simulink model "s0416"  (Simulink 7.0)
settings: Solver=ode3  SolverMode=SingleTasking  StartTime=0.0  StopTime=900  FixedStep=1  MaxStep=1  RelTol=1e-3  AbsTol=1e-6
values from neighbouring files (symbols this model uses):
  Kpr = 10    [m0108d.m]    (also in m0109b.m = 1; m0113c.m; m0404Bsp.m = 3)
  t0A = -1    [m0404Bsp.m]
undefined symbols (not defined in the file or in its folder): eAdach, edach, T1D, Tv
settings Model: Creator=froriep  LastModifiedBy=froriep
settings DataIOCC: LimitDataPoints=off  SaveOutput=off  SaveTime=off
settings OptimizationCC: BooleanDataType=off
settings DebuggingCC: SaveWithParameterizedLinksMsg=none  SignalResolutionControl=TryResolveAllWithWarning  SolverPrmCheckMsg=none  MultiTaskDSMMsg=warning  MultiTaskCondExecSysMsg=none  StrictBusMsg=None
settings HardwareCC: TargetUnknown=on
settings RTWCC: IncludeERTFirstTime=on

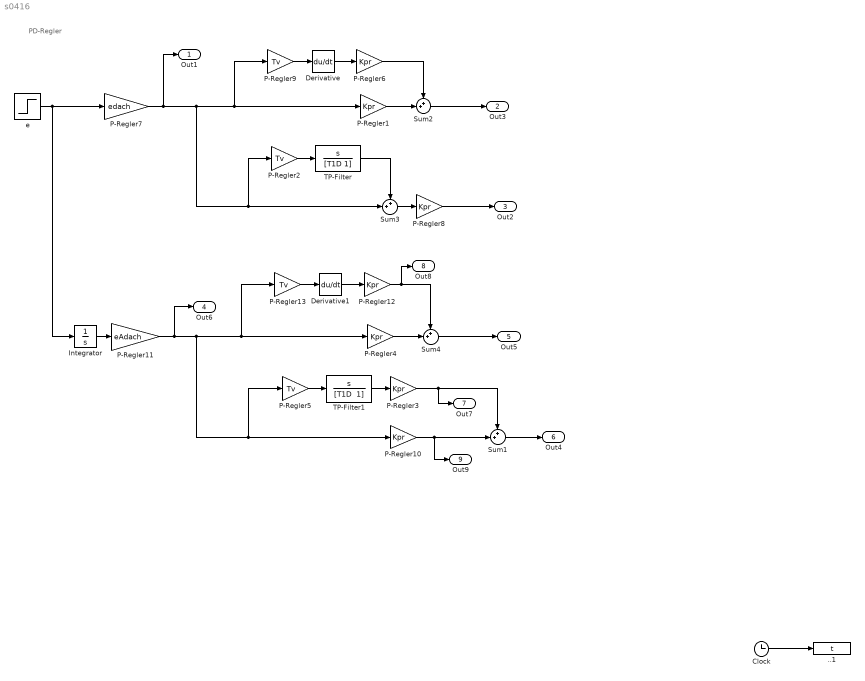
== system s0416 ==
  note: PD-Regler
  ..1 : ToWorkspace  VariableName=t  SaveFormat=Array
  Clock : Clock
      settings: Decimation=10
  Derivative : Derivative
  Derivative1 : Derivative
  Integrator : Integrator
  P-Regler{1,3..4,6,8,10,12} (7 alike) : Gain  Gain=Kpr  ParameterDataType=sfix(16)  ParameterScaling=2^0  OutDataType=sfix(16)  OutScaling=2^0
  P-Regler11 : Gain  Gain=eAdach  ParameterDataType=sfix(16)  ParameterScaling=2^0  OutDataType=sfix(16)  OutScaling=2^0
  P-Regler{2,5,9,13} (4 alike) : Gain  Gain=Tv  ParameterDataType=sfix(16)  ParameterScaling=2^0  OutDataType=sfix(16)  OutScaling=2^0
  P-Regler7 : Gain  Gain=edach  ParameterDataType=sfix(16)  ParameterScaling=2^0  OutDataType=sfix(16)  OutScaling=2^0
  Sum{1..4} (4 alike) : Sum  Inputs=++|  SaturateOnIntegerOverflow=on  InputSameDT=on
  TP-Filter : TransferFcn  Numerator=[1 0]  Denominator=[T1D 1]
  TP-Filter1 : TransferFcn  Numerator=[1 0]  Denominator="[T1D  1]"
  e : Step  Time=-t0A  SampleTime=0
  Out1 : Outport  OutDataType=sfix(16)  OutScaling=2^0
  Out3 : Outport  Port=2  OutDataType=sfix(16)  OutScaling=2^0
  Out2 : Outport  Port=3  OutDataType=sfix(16)  OutScaling=2^0
  Out6 : Outport  Port=4  OutDataType=sfix(16)  OutScaling=2^0
  Out5 : Outport  Port=5  OutDataType=sfix(16)  OutScaling=2^0
  Out4 : Outport  Port=6  OutDataType=sfix(16)  OutScaling=2^0
  Out7 : Outport  Port=7  OutDataType=sfix(16)  OutScaling=2^0
  Out8 : Outport  Port=8  OutDataType=sfix(16)  OutScaling=2^0
  Out9 : Outport  Port=9  OutDataType=sfix(16)  OutScaling=2^0
  wires:
  e/1 -> P-Regler7/1, Integrator/1
  Clock/1 -> ..1/1
  Sum3/1 -> P-Regler8/1
  P-Regler2/1 -> TP-Filter/1
  TP-Filter/1 -> Sum3/1
  Integrator/1 -> P-Regler11/1
  Sum1/1 -> Out4/1
  P-Regler5/1 -> TP-Filter1/1
  TP-Filter1/1 -> P-Regler3/1
  P-Regler7/1 -> Out1/1, P-Regler2/1, Sum3/2, P-Regler1/1, P-Regler9/1
  P-Regler8/1 -> Out2/1
  P-Regler3/1 -> Sum1/1, Out7/1
  P-Regler10/1 -> Sum1/2, Out9/1
  P-Regler11/1 -> P-Regler5/1, P-Regler10/1, P-Regler4/1, P-Regler13/1, Out6/1
  P-Regler9/1 -> Derivative/1
  Derivative/1 -> P-Regler6/1
  P-Regler1/1 -> Sum2/2
  P-Regler6/1 -> Sum2/1
  Sum2/1 -> Out3/1
  P-Regler13/1 -> Derivative1/1
  Derivative1/1 -> P-Regler12/1
  P-Regler12/1 -> Sum4/1, Out8/1
  P-Regler4/1 -> Sum4/2
  Sum4/1 -> Out5/1
